simulink model "graycode"  (Simulink 6.0)
settings: Solver=ode45  SolverMode=SingleTasking  StartTime=0.0  StopTime=inf  RelTol=1e-3  AbsTol=1e-6
PreLoadFcn:
  | EbNo=3;maxNumErrs=100;maxNumBits=1e8;M=8;Tsample=.01;Tsym=.2;
model workspace: external: M-Code (data not in the file)
undefined symbols (not defined in the file or in its folder): slcm
libraries: commutil2 x2, commsink2 x2, commdigbbndpm2 x2, commchan2 x1, commrandsrc2 x1
CloseFcn:
  | clear graySER grayBER graySigsOut EbNo maxNumErrs maxNumBits M Tsample Tsym
settings Model: RequirementInfo=9  CovMetricSettings=d  Creator=tdelve  LastModifiedBy=ysong  ExtModeTrigMode=oneshot  ExtModeArmWhenConnect=off  ExtModeAutoUpdateStatusClock=off  ProdHWDeviceType=Specified
settings DataIOCC: LimitDataPoints=off  SaveOutput=off  SaveTime=off  SignalLoggingName=graySigsOut
settings OptimizationCC: BlockReduction=off  BooleanDataType=off
settings DebuggingCC: CheckExecutionContextPreStartOutputMsg=on  CheckExecutionContextRuntimeOutputMsg=on  SolverPrmCheckMsg=none  IntegerOverflowMsg=none
settings HardwareCC: ProdHWDeviceType=Specified
settings ModelReferenceCC: UpdateModelReferenceTargets=IfOutOfDate
settings CodeAppCC: MangleLength=5
settings GRTTargetCC: LifeSpan=inf
settings SFSimCC: SFSimApplyToAllLibs=on  SFSimBuildMode=Incremental

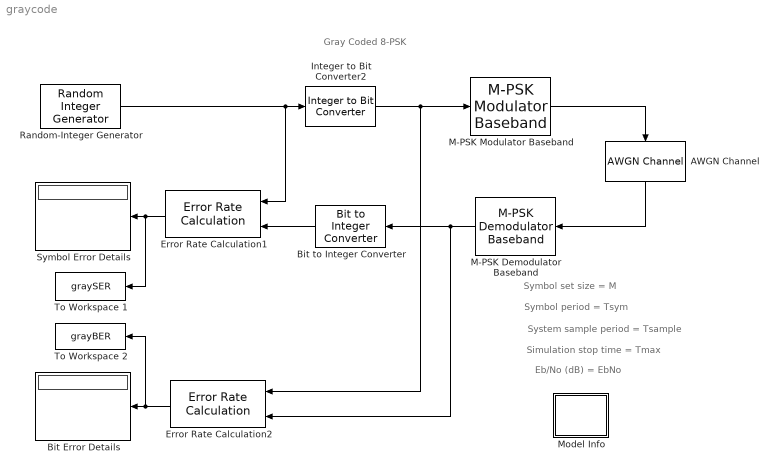
== system graycode ==
  note: Gray Coded 8-PSK
  note: Symbol set size = M
  note: Symbol period = Tsym
  note: System sample period = Tsample
  note: Eb/No (dB) = EbNo
  note: Simulation stop time = Tmax
  AWGN Channel : commchan2/AWGN Channel  Orientation=down  seed=67  noiseMode="Signal to noise ratio  (Eb/No)"  EbNodB=EbNo  EsNodB=EbNo+10*log10(log2(M))  SNRdB=10  bitsPerSym=log2(M)  Ps=1  Tsym=Tsym  variance=1
  Bit Error Details : Display
  Bit to Integer Converter : commutil2/Bit to Integer Converter  Orientation=left  nbits=log2(M)
  Error Rate Calculation1 : commsink2/Error Rate Calculation  Orientation=left  N=0  st_delay=0  cp_mode=Entire frame  subframe=[]  PMode=Port  WsName=SymErrorVec  RsMode2=off  stop=off  numErr=100  maxBits=1e6
  Error Rate Calculation2 : commsink2/Error Rate Calculation  Orientation=left  N=0  st_delay=0  cp_mode=Entire frame  subframe=[]  PMode=Port  WsName=BitErrorVec  RsMode2=off  stop=on  numErr=maxNumErrs  maxBits=maxNumBits
  Integer to Bit Converter2 : commutil2/Integer to Bit Converter  nbits=log2(M)
  M-PSK Demodulator Baseband : commdigbbndpm2/M-PSK Demodulator Baseband  Orientation=left  M=M  OutType=Bit  Dec=Gray  Ph=0  numSamp=1
  M-PSK Modulator Baseband : commdigbbndpm2/M-PSK Modulator Baseband  M=M  InType=Bit  Enc=Gray  Ph=0  numSamp=1
  Model Info : Subsystem  LoadFcn=slcm LoadBlock;  InitFcn=slcm('UpdateAllCMBlocksInThisModelInit')  EnableExecutionContextPropagation=on  mask(CMBlock){InitialSaveTempField=, InitialBlockCM=none, BlockCM=none, Frame=on, SaveTempField=, DisplayStringWithTags=Info, MaskDisplayString=Info, HorizontalTextAlignment=Center, LeftAlignmentValue=0.5, SourceBlockDiagram=graycode, TagMaxNumber=20, CMTag1=, CMTag2=, CMTag3=, CMTag4=, CMTag5=, CMTag6=, CMTag7=, CMTag8=, CMTag9=, CMTag10=, CMTag11=, CMTag12=, CMTag13=, CMTag14=, CMTag15=, CMTag16=, CMTag17=, CMTag18=, CMTag19=, CMTag20=}
      mask help: This block allows revision control information to be displayed within the model.
      settings: CopyFcn=slcm CopyBlock;  DeleteFcn=slcm Cancel;  PostSaveFcn=slcm('UpdateAllCMBlocksInThisModel')  NameChangeFcn=slcm Rename;  OpenFcn=commdemohelp;
      mask Display: text(str2num(LeftAlignmentValue), 0.5, MaskDisplayString, 'HorizontalAlignment', HorizontalTextAlignment)
  Random-Integer Generator : commrandsrc2/Random Integer Generator  mul=M  seed=529558  Ts=Tsym  frameBased=on  sampPerFrame=100  orient=off
  Symbol Error Details : Display
  To Workspace 1 : ToWorkspace  VariableName=graySER  SampleTime=-1  SaveFormat=Array
      settings: MaxDataPoints=1
  To Workspace 2 : ToWorkspace  VariableName=grayBER  SampleTime=-1  SaveFormat=Array
      settings: MaxDataPoints=1
  wires:
  Error Rate Calculation2/1 -> Bit Error Details/1, To Workspace 2/1
  Error Rate Calculation1/1 -> Symbol Error Details/1, To Workspace 1/1
  M-PSK Demodulator Baseband/1 -> Bit to Integer Converter/1, Error Rate Calculation2/2
  Random-Integer Generator/1 -> Integer to Bit Converter2/1, Error Rate Calculation1/1
  AWGN Channel/1 -> M-PSK Demodulator Baseband/1
  M-PSK Modulator Baseband/1 -> AWGN Channel/1
  Integer to Bit Converter2/1 -> M-PSK Modulator Baseband/1, Error Rate Calculation2/1
  Bit to Integer Converter/1 -> Error Rate Calculation1/2

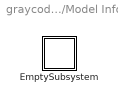
== system graycode/Model Info ==
  EmptySubsystem : Subsystem  EnableExecutionContextPropagation=on

== system graycode/Model Info/EmptySubsystem ==
